simulink model "mealy"  (R2015a)
settings: Solver=ode3  StartTime=0.0  StopTime=10  FixedStep=1  RelTol=1e-3
undefined symbols (not defined in the file): sigbuilder_block
settings Model: Creator=Student  LastModifiedBy=lenovo

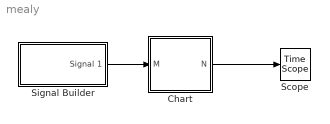
== system mealy ==
  Chart : Stateflow chart  TreatAsAtomicUnit=on
  Scope : TimeScope
  Signal Builder : Subsystem  Tag=STV Subsys  LoadFcn=sigbuilder_block('load');  StartFcn=sigbuilder_block('start');  StopFcn=sigbuilder_block('stop');  ClipboardFcn=sigbuilder_block('clipboard');  mask(Sigbuilder block){}
      mask help: Simulink:masks:SigbuilderBlock_MD
      mask init:
      | if ~strcmp(get_param(bdroot(gcbh),'SimulationStatus'),'stopped') tuvar = sigbuilder_block('maskInit'); end
      settings: CopyFcn=sigbuilder_block('copy');  DeleteFcn=sigbuilder_block('delete');  ModelCloseFcn=sigbuilder_block('modelClose');  PreSaveFcn=sigbuilder_block('preSave');  PauseFcn=sigbuilder_block('pause');  ContinueFcn=sigbuilder_block('continue');  NameChangeFcn=sigbuilder_block('namechange');  OpenFcn=sigbuilder_block('open',[437.6 199.2 550.4 400 ]);  CloseFcn=sigbuilder_block('close');
      mask Display: plot(0, 0, 100, 100,[2, 2, 32, 32, 2], [68, 8, 8, 68, 68],[32, 2], [38, 38], [32, 19, 2],[53, 60, 44], [32, 17, 17, 2],[16, 16, 31, 31]);txt = getActiveGroup(gcbh);text(2, 100, txt,'verticalAlignment', 'top');
  wires:
  Chart/1(N) -> Scope/1
  Signal Builder/1(Signal 1) -> Chart/1(M)

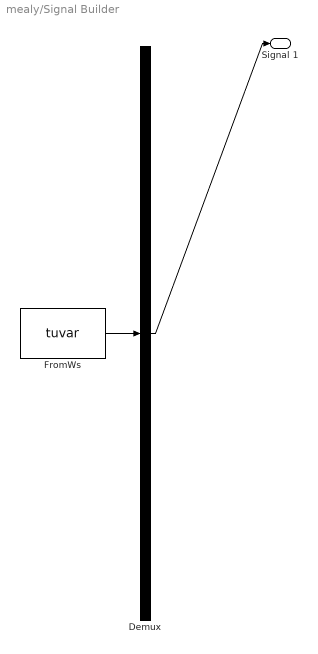
== system mealy/Signal Builder ==
  Demux : Demux  Tag=STV Demux  Outputs=1
  FromWs : FromWorkspace  Tag=STV FromWs  VariableName=tuvar  SampleTime=0
      SigBuilderData=|
      | common.afterFinalStr = 'Extrapolate'
      | common.sampleTime = 0
      | dataSet.timeRange = [0 10]
      | dataSet.name = 'Group 1'
      | sbobj.Groups.Name = 'Group 1'
      | sbobj.Groups.Signals.Name = 'Signal 1'
      | sbobj.Groups.Signals.XData = [0 1 2 2 2.14 2.14 4 4 4.18 4.18 6 6 6.16 6.16 8 8 8.2 8.2 10]
      | sbobj.Groups.Signals.YData = [0 0 0 1 1 0 0 2 2 0 0 1 1 0 0 2 2 0 0]
  Signal 1 : Outport  Tag=STV Outport
  wires:
  FromWs/1 -> Demux/1
  Demux/1 -> Signal 1/1

== stateflow chart mealy/Chart ==
  settings: stateMachineType=MEALY_MACHINE
  state jeden
  state zero
  state dwa
  (default) -> zero [order 2]
  zero -> jeden [order 1] : [M==1]{N=0}
  jeden -> zero : [M==2]{N=1}
  dwa -> jeden [order 1] : [M==2]{N=1}
  zero -> dwa [order 2] : [M==2]{N=0}
  dwa -> zero [order 3] : [M==1]{N=1}
  (default) -> dwa [order 1] : [M==1]{N=0}
  dwa -> dwa [order 2] : [M==2]{N=1}
  data: M input; N output
